simulink model "chap4_6sim"  (Simulink 6.3)
settings: Solver=ode5  StartTime=0.0  StopTime=10  FixedStep=0.001  RelTol=1e-3
settings Model: Creator=hp  LastModifiedBy=Administrator
settings DebuggingCC: SolverPrmCheckMsg=none

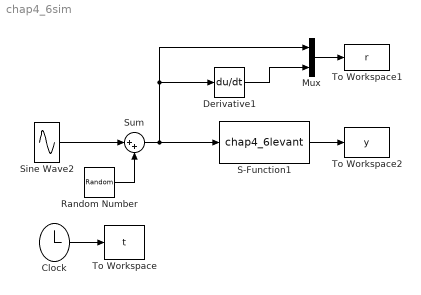
== system chap4_6sim ==
  Clock : Clock
      settings: Decimation=30
  Derivative1 : Derivative
  Mux : Mux  Inputs=2
  Random Number : RandomNumber  Variance=0.01  SampleTime=0
  S-Function1 : S-Function  FunctionName=chap4_6levant
  Sine Wave2 : Sin  SampleTime=0
  Sum : Sum  Inputs=|++
  To Workspace : ToWorkspace  VariableName=t  SampleTime=-1  SaveFormat=Array
  To Workspace1 : ToWorkspace  VariableName=r  SampleTime=-1  SaveFormat=Array
  To Workspace2 : ToWorkspace  VariableName=y  SampleTime=-1  SaveFormat=Array
  wires:
  Clock/1 -> To Workspace/1
  S-Function1/1 -> To Workspace2/1
  Sine Wave2/1 -> Sum/1
  Random Number/1 -> Sum/2
  Sum/1 -> S-Function1/1, Mux/1, Derivative1/1
  Mux/1 -> To Workspace1/1
  Derivative1/1 -> Mux/2
